simulink model "testDynamics"  (R2021a)
settings: Solver=VariableStepAuto  StartTime=0.0  StopTime=Torb  RelTol=1e-3
libraries: sharedtransform x3, aerolibutil x2
settings Model: Creator=Laura  LastModifiedBy=Laura

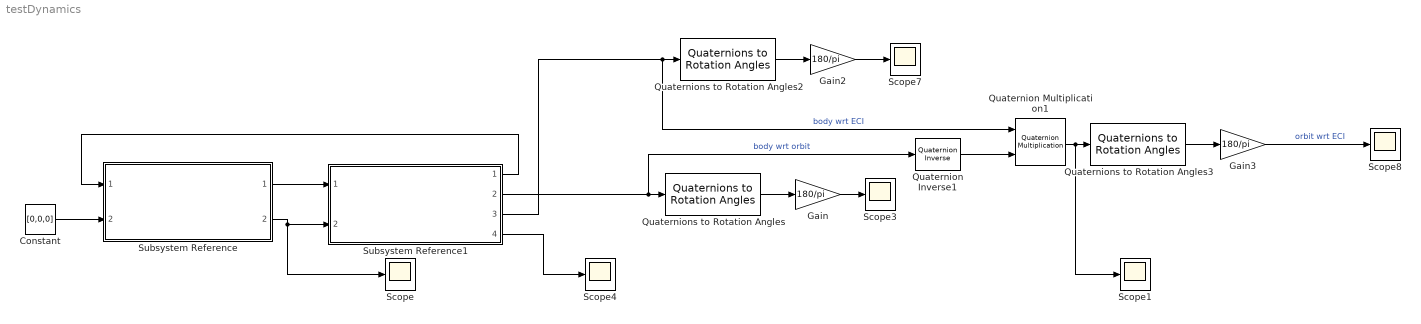
== system testDynamics ==
  Constant : Constant  Value=[0,0,0]
  Gain : Gain  Gain=180/pi
  Gain2 : Gain  Gain=180/pi
  Gain3 : Gain  Gain=180/pi
  Quaternion Inverse1 : aerolibutil/Quaternion Inverse
  Quaternion Multiplication1 : aerolibutil/Quaternion Multiplication
  Quaternions to Rotation Angles : sharedtransform/Quaternions to Rotation Angles  rotationOrder=ZYX  aMode=aMode
      settings: SourceProductBaseCode=AE,PW,DR,MT,UV,VE
  Quaternions to Rotation Angles2 : sharedtransform/Quaternions to Rotation Angles  rotationOrder=ZYX  aMode=aMode
      settings: SourceProductBaseCode=AE,PW,DR,MT,UV,VE
  Quaternions to Rotation Angles3 : sharedtransform/Quaternions to Rotation Angles  rotationOrder=ZYX  aMode=aMode
      settings: SourceProductBaseCode=AE,PW,DR,MT,UV,VE
  Scope{,1,3..4,7..8} (6 alike) : Scope
  Subsystem Reference : Subsystem  ReferencedSubsystem=Dynamics
  Subsystem Reference1 : Subsystem  ReferencedSubsystem=Kinematics
  wires:
  Subsystem Reference1/1 -> Subsystem Reference/1
  Subsystem Reference/2 -> Scope/1, Subsystem Reference1/2
  Subsystem Reference/1 -> Subsystem Reference1/1
  Constant/1 -> Subsystem Reference/2
  Quaternions to Rotation Angles/1 -> Gain/1
  Gain/1 -> Scope3/1
  Quaternions to Rotation Angles2/1 -> Gain2/1
  Gain2/1 -> Scope7/1
  Subsystem Reference1/3 -> Quaternion Multiplication1/1, Quaternions to Rotation Angles2/1  "body wrt ECI"
  Quaternion Inverse1/1 -> Quaternion Multiplication1/2
  Gain3/1 -> Scope8/1  "orbit wrt ECI"
  Quaternions to Rotation Angles3/1 -> Gain3/1
  Quaternion Multiplication1/1 -> Scope1/1, Quaternions to Rotation Angles3/1
  Subsystem Reference1/2 -> Quaternion Inverse1/1, Quaternions to Rotation Angles/1  "body wrt orbit"
  Subsystem Reference1/4 -> Scope4/1
